simulink model "newautotest"  (R2021a)
settings: Solver=FixedStepAuto  StartTime=0.0  StopTime=inf  RelTol=1e-3  EnableMultiTasking=on
libraries: vexarmcortexlib x4
settings Model: ExtModeTrigDuration=25  Creator=Mihai Nicoara  LastModifiedBy=Mihai Nicoara
settings OptimizationCC: EnhancedBackFolding=on  PassReuseOutputArgsAs=Individual arguments  ZeroExternalMemoryAtStartup=off  ZeroInternalMemoryAtStartup=off  MaxStackSize=64  OptimizeBlockOrder=speed  DifferentSizesBufferReuse=on  OptimizationCustomize=off  EfficientTunableParamExpr=on
settings DebuggingCC: ParameterTunabilityLossMsg=error
settings HardwareCC: ProdBitPerPointer=32  ProdBitPerSizeT=32  ProdBitPerPtrDiffT=32  ProdLargestAtomicInteger=Long  ProdLargestAtomicFloat=Double  ProdWordSize=32  ProdHWDeviceType=ARM Compatible->ARM Cortex
settings SFSimCC: MATLABDynamicMemAlloc=off
settings RTWCC: SystemTargetFile=ert.tlc  HardwareBoard=ARM Cortex-based VEX Microcontroller  TLCOptions="-aInlineSetEventsForThisBaseRateFcn=TLC_FALSE -aSuppressMultiTaskScheduler=TLC_FALSE  -aRateBasedStepFcn=0"  TemplateMakefile=ert_default_tmf  Toolchain=GNU Tools for VEX ARM Cortex
settings CodeAppCC: ForceParamTrailComments=on  IgnoreCustomStorageClasses=off  OperatorAnnotations=on  SimulinkDataObjDesc=on  SFDataObjDesc=on  InsertBlockDesc=on
settings ERTTargetCC: ExtModeTransport=1  ExtModeMexFile=ext_serial_win32_comm

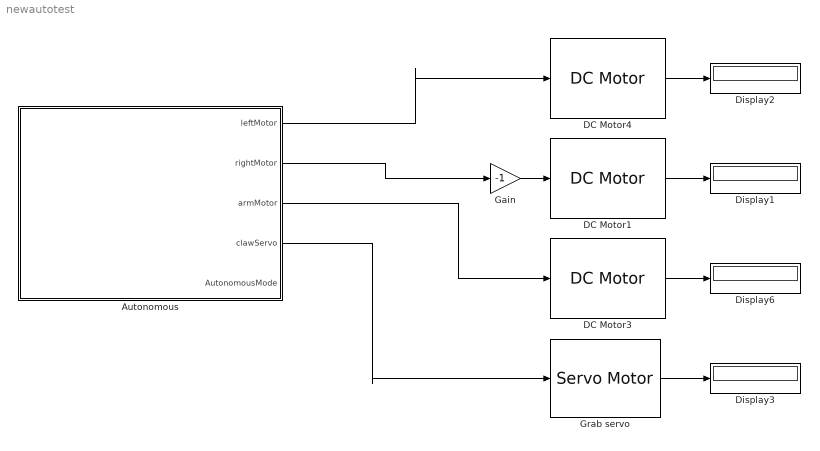
== system newautotest ==
  Autonomous : Stateflow chart  TreatAsAtomicUnit=on
  DC Motor1 : vexarmcortexlib/Actuators/DC Motor  motor=2  scaleFactor=1/13.5  SimulationOut=on
      settings: SourceProductBaseCode=EC_VEX_MICRO
  DC Motor3 : vexarmcortexlib/Actuators/DC Motor  motor=7  scaleFactor=1/13.5  SimulationOut=on
      settings: SourceProductBaseCode=EC_VEX_MICRO
  DC Motor4 : vexarmcortexlib/Actuators/DC Motor  motor=9  scaleFactor=1/13.5  SimulationOut=on
      settings: SourceProductBaseCode=EC_VEX_MICRO
  Display{1..3,6} (4 alike) : Display
  Gain : Gain  Gain=-1
  Grab servo : vexarmcortexlib/Actuators/Servo Motor  motor=3  scaleFactor=60/127  SimulationOut=on
      settings: SourceProductBaseCode=EC_VEX_MICRO
  wires:
  Gain/1 -> DC Motor1/1
  DC Motor1/1 -> Display1/1
  Autonomous/2(rightMotor) -> Gain/1
  DC Motor4/1 -> Display2/1
  Autonomous/1(leftMotor) -> DC Motor4/1
  DC Motor3/1 -> Display6/1
  Autonomous/3(armMotor) -> DC Motor3/1
  Grab servo/1 -> Display3/1
  Autonomous/4(clawServo) -> Grab servo/1

== stateflow chart newautotest/Autonomous ==
  state Start
    entry:
    leftMotor = 0;
    rightMotor = 0;
    armMotor = 0;
    clawServo = 0;
  state A
    entry:
    leftMotor = 0;
    rightMotor = 0;
    armMotor = -40;
  state B
    entry:
    leftMotor = -100;
    rightMotor = -100;
    armMotor = 0;
  state E
    entry:
    leftMotor = 0;
    rightMotor = 0;
    armMotor = 40;
  state C
    entry:
    leftMotor = 0;
    rightMotor = 0;
    armMotor = 0;
  state D
    entry:
    leftMotor = 100;
    rightMotor = 100;
    armMotor = 0;
  state F
    entry:
    leftMotor = 0;
    rightMotor = 0;
    armMotor =  0;
    clawServo = 200;
  state G
    entry:
    leftMotor = 0;
    rightMotor = 0;
    armMotor =  40;
    clawServo = 200;
  state H
    entry:
    leftMotor = -100;
    rightMotor = -100;
    armMotor =  -40;
    clawServo = 200;
  state I
    entry:
    leftMotor = 0;
    rightMotor = 0;
    armMotor =  0;
    clawServo = 200;
  (default) -> Start
  Start -> A : [after(1,sec)]
  A -> B : [after(1,sec)]
  I -> Start : [after(5,sec)]
  B -> C : [after(1, sec)]
  C -> D : [after(1,sec)]
  D -> E : [after(1,sec)]
  E -> F : [after(1,sec)]
  F -> G : [after(1,sec)]
  G -> H : [after(1,sec)]
  H -> I : [after(1,sec)]
  data: leftMotor output; rightMotor output; armMotor output; clawServo output; AutonomousMode output Enum: AutonomousModeType
